simulink library "EngineModelsLibrary"  (R2014b)
settings: Solver=ode45  StartTime=0.0  StopTime=10.0  RelTol=1e-3
values from neighbouring files (symbols this model uses):
  k = 0.2    [ES_Run.m]    (also in ES_Run_v2.m = 10)
undefined symbols (not defined in the file or in its folder): b, COBRA_Compressor, cp, CPT_COBRA_LIB, D, etalim, gam, Newton, Pa, PARAM, Pl, pref, Ps, R, Raphson, rlim, T_0, Tref, Wclim
undefined symbols (not defined in the file): cr, e, etagain, fit_pars, kL, kS, par
(part 2 of 3)

== system EngineModelsLibrary/Throttle [Alt] ==
  pin (Pa) : Inport
  Tin (K) : Inport  Port=2
  pout (Pa) : Inport  Port=3
  Tout (K) : Inport  Port=4
  uth (%) : Inport  Port=5
  Compressible flow : Subsystem  mask{gam=gam, R=R, PIlin=PIlin}
      mask prompts: gam "Specific heat ratio (-)"; R "Ideal gas constant (J/kg/K)"; PIlin "Linear segment minimum pressure ratio (-)"
      mask help: Isentropic compressible flow, see App. C in Heywood (1988). Modified by adding a linear segment for pressure ratios larger than the parameter PIlin. In this way, it is possible to avoid infinite derivative for pressure ratios close to one. -- erikhe@umich
  Throttle area : Subsystem
  Wth (kg/s) : Outport
  Tth (K) : Outport  Port=2
  wires:
  uth (%)/1 -> Throttle area/1(uth (%))
  pin (Pa)/1 -> Compressible flow/1(pin (Pa))
  Tin (K)/1 -> Compressible flow/2(Tin (K))
  pout (Pa)/1 -> Compressible flow/3(pout (Pa))
  Tout (K)/1 -> Compressible flow/4(Tout (K))
  Throttle area/1(A (m^2)) -> Compressible flow/5(Aeff (m^2))
  Compressible flow/1(mflow (kg/s)) -> Wth (kg/s)/1
  Compressible flow/2(Tflow (K)) -> Tth (K)/1

== system EngineModelsLibrary/Throttle [simple] ==
  pin (Pa) : Inport
  Tin (K) : Inport  Port=2
  pout (Pa) : Inport  Port=3
  Tout (K) : Inport  Port=4
  uth (-) : Inport  Port=5
  Compressible flow : Subsystem  mask{gam=gam, R=R, PIlin=PIlin}
      mask prompts: gam "Specific heat ratio (-)"; R "Ideal gas constant (J/kg/K)"; PIlin "Linear segment minimum pressure ratio (-)"
      mask help: Isentropic compressible flow, see App. C in Heywood (1988). Modified by adding a linear segment for pressure ratios larger than the parameter PIlin. In this way, it is possible to avoid infinite derivative for pressure ratios close to one. -- erikhe@umich
  Gain : Gain  Gain=pi
  Throttle area : Subsystem
  Wth (kg/s) : Outport
  Tth (K) : Outport  Port=2
  wires:
  Compressible flow/2(Tflow (K)) -> Tth (K)/1
  Compressible flow/1(mflow (kg/s)) -> Wth (kg/s)/1
  Throttle area/1(A (m^2)) -> Compressible flow/5(Aeff (m^2))
  Tout (K)/1 -> Compressible flow/4(Tout (K))
  pout (Pa)/1 -> Compressible flow/3(pout (Pa))
  Tin (K)/1 -> Compressible flow/2(Tin (K))
  pin (Pa)/1 -> Compressible flow/1(pin (Pa))
  Gain/1 -> Throttle area/1(alpha (rad))
  uth (-)/1 -> Gain/1

== system EngineModelsLibrary/Turbine [Eriksson] ==
  pin (Pa) : Inport
  Tin (K) : Inport  Port=2
  w (rad/s) : Inport  Port=3
  pout (Pa) : Inport  Port=4
  Efficiency : Subsystem
  Mass flow : Subsystem
  Power : Subsystem
  Pressure ratio w saturation : Subsystem
  Temperature : Subsystem
  To Workspace2 : ToWorkspace  VariableName=etat  SampleTime=-1
  Tt (K) : Outport
  Wt (kg/s) : Outport  Port=2
  Pt (W) : Outport  Port=3
  wires:
  Power/1(P (W)) -> Pt (W)/1
  Pressure ratio w saturation/1(PI (-)) -> Mass flow/3(PI (-)), Efficiency/1(PI (-)), Temperature/1(PI (-))
  Tin (K)/1 -> Mass flow/2(Tin (K)), Efficiency/2(Tin (K)), Temperature/2(Tin (K)), Power/2(Tin (K))
  w (rad/s)/1 -> Efficiency/3(w (rad/s))
  Efficiency/1(etat (-)) -> To Workspace2/1, Temperature/3(etat (-))
  Temperature/1(Tout (K)) -> Power/3(Tout (K)), Tt (K)/1
  Mass flow/1(Wt (kg/s)) -> Power/1(W (kg/s)), Wt (kg/s)/1
  pin (Pa)/1 -> Mass flow/1(pin (Pa)), Pressure ratio w saturation/1(pin (Pa))
  pout (Pa)/1 -> Pressure ratio w saturation/2(pout (Pa))

== system EngineModelsLibrary/Turbine [Jensen,Moraal] ==
  pin (Pa) : Inport
  Tin (K) : Inport  Port=2
  w (rad/s) : Inport  Port=3
  pout (Pa) : Inport  Port=4
  Corrected speed : Subsystem
  Efficiency : Subsystem
  Gain : Gain  Gain=60
  Mass flow : Subsystem
  Power : Subsystem
  Pressure ratio w saturation : Subsystem
  Temperature : Subsystem
  Pt (W) : Outport
  etat (-) : Outport  Port=2
  Tt (K) : Outport  Port=3
  Wt (kg/s) : Outport  Port=4
  wires:
  w (rad/s)/1 -> Corrected speed/2(w (rad/s))
  Tin (K)/1 -> Corrected speed/1(Tin (K)), Mass flow/2(Tin (K)), Power/2(Tin (K)), Temperature/2(Tin (K))
  pin (Pa)/1 -> Mass flow/1(pin (Pa)), Pressure ratio w saturation/1(pin (Pa))
  pout (Pa)/1 -> Pressure ratio w saturation/2(pout (Pa))
  Pressure ratio w saturation/1(PI (-)) -> Temperature/1(PI (-)), Efficiency/1(PI (-)), Mass flow/3(PI (-))
  Corrected speed/1(Nc corr (rps/K^.5)) -> Gain/1
  Mass flow/1(Wt (kg/s)) -> Wt (kg/s)/1, Power/1(W (kg/s))
  Temperature/1(Tout (K)) -> Tt (K)/1, Power/3(Tout (K))
  Efficiency/1(etat (-)) -> etat (-)/1, Temperature/3(etat (-))
  Power/1(P (W)) -> Pt (W)/1
  Gain/1 -> Mass flow/4(Ncorr (rpm/K^.5)), Efficiency/2(Ncorr (rpm/K^.5))

== system EngineModelsLibrary/Turbine and wastegate ==
  note: Wastegate is a compressible flow restriction. Flows are assumed to be mixed
      | adiabatically with constant specific heat (i.e., mass-averaged temperature).
      | -- erikhe@umich
  pin (Pa) : Inport
  w (rad/s) : Inport  Port=2
  Tin (K) : Inport  Port=3
  pout (Pa) : Inport  Port=4
  uwg (%) : Inport  Port=5
  Gain : Gain  Gain=PARAM.wastegate.C
  Product : Product  RndMeth=Zero
  Product1 : Product  RndMeth=Zero
  Product2 : Product  Inputs=*/  RndMeth=Zero
  Saturation : Saturate  UpperLimit=100  LowerLimit=0
  Sum : Sum  Inputs=++|
  Sum1 : Sum
  Turbine [Jensen,Moraal] : Subsystem  mask{gam=PARAM.exh.gamma, cp=PARAM.exh.cp, D=PARAM.turbine.D, k11=PARAM.turbine.k11, k12=PARAM.turbine.k12, k21=PARAM.turbine.k21, k22=PARAM.turbine.k22, PIlin=PARAM.turbine.PIlin, Wtcmax=PARAM.turbine.Wtcmax, Wtcmin=PARAM.turbine.Wtcmin, b0=PARAM.turbine.b0, b1=PARAM.turbine.b1, b2=PARAM.turbine.b2, b3=PARAM.turbine.b3, b4=PARAM.turbine.b4, b5=PARAM.turbine.b5, etamax=PARAM.turbine.etamax, etamin=PARAM.turbine.etamin}
      mask prompts: gam "Ratio of specific heats (-)"; cp "Specific heat cp (J/kg/K)"; D "Diameter (m)"; k11 "Mass flow fit k11"; k12 "Mass flow fit k12"; k21 "Mass flow fit k21"; k22 "Mass flow fit k22"; PIlin "Mass flow PIlin"; Wtcmax "Mass flow max (kg/s K^.5/Pa)"; Wtcmin "Mass flow min (kg/s K^.5/Pa)"; b0 "Efficiency fit b0"; b1 "Efficiency fit b1"; b2 "Efficiency fit b2"; b3 "Efficiency fit b3"; b4 "Efficiency fit b4"; b5 "Efficiency fit b5"; etamax "Efficiency max (-)"; etamin "Efficiency min (-)"
  Wastegate : Subsystem  mask{gam=PARAM.exh.gamma, R=PARAM.exh.R, PIlin=PARAM.wastegate.PIlin}
      mask prompts: gam "Specific heat ratio (-)"; R "Ideal gas constant (J/kg/K)"; PIlin "Linear segment minimum pressure ratio (-)"
      mask help: Isentropic compressible flow, see App. C in Heywood (1988). Modified by adding a linear segment for pressure ratios larger than the parameter PIlin. In this way, it is possible to avoid infinite derivative for pressure ratios close to one. -- erikhe@umich
  Tout  (K) : Outport
  Wt (kg/s) : Outport  Port=2
  Wwg (kg/s) : Outport  Port=3
  Pt (W) : Outport  Port=4
  etat (-) : Outport  Port=5
  wires:
  Saturation/1 -> Gain/1
  Product2/1 -> Tout  (K)/1
  Sum1/1 -> Product2/1
  Product1/1 -> Sum1/2
  Product/1 -> Sum1/1
  Wastegate/2(Tflow (K)) -> Product1/2
  Turbine [Jensen,Moraal]/3(Tt (K)) -> Product/1
  Turbine [Jensen,Moraal]/4(Wt (kg/s)) -> Wt (kg/s)/1, Sum/1, Product/2
  Turbine [Jensen,Moraal]/1(Pt (W)) -> Pt (W)/1
  Turbine [Jensen,Moraal]/2(etat (-)) -> etat (-)/1
  Sum/1 -> Product2/2
  Wastegate/1(mflow (kg/s)) -> Wwg (kg/s)/1, Product1/1, Sum/2
  Gain/1 -> Wastegate/4(Aeff (m^2))
  uwg (%)/1 -> Saturation/1
  pout (Pa)/1 -> Wastegate/3(pout (Pa)), Turbine [Jensen,Moraal]/4(pout (Pa))
  w (rad/s)/1 -> Turbine [Jensen,Moraal]/3(w (rad/s))
  Tin (K)/1 -> Wastegate/2(Tin (K)), Turbine [Jensen,Moraal]/2(Tin (K))
  pin (Pa)/1 -> Wastegate/1(pin (Pa)), Turbine [Jensen,Moraal]/1(pin (Pa))

== system EngineModelsLibrary/Twin-Scroll Turbine ==
  Pems (Pa) : Inport
  Peml (Pa) : Inport  Port=2
  Pex (Pa) : Inport  Port=3
  omega (rad/s) : Inport  Port=4
  Tems (K) : Inport  Port=5
  Teml (K) : Inport  Port=6
  Demux : Demux  Outputs=5
  Mux : Mux  Inputs=6
  S-Function : S-Function  FunctionName=turbine  Parameters=eta,gam,cp,smar_fit,smar_lim,flow_fit,flow_lim  SFunctionModules=turbine engine_model  EnableBusSupport=off
  Power (W) : Outport
  Wtl (kg/s) : Outport  Port=2
  Wts (kg/s) : Outport  Port=3
  Temp (K) : Outport  Port=4
  SMaR (-) : Outport  Port=5
  wires:
  Demux/1 -> Power (W)/1
  Pems (Pa)/1 -> Mux/1
  Peml (Pa)/1 -> Mux/2
  Pex (Pa)/1 -> Mux/3
  omega (rad/s)/1 -> Mux/4
  Mux/1 -> S-Function/1
  S-Function/1 -> Demux/1
  Demux/2 -> Wtl (kg/s)/1
  Tems (K)/1 -> Mux/5
  Teml (K)/1 -> Mux/6
  Demux/3 -> Wts (kg/s)/1
  Demux/4 -> Temp (K)/1
  Demux/5 -> SMaR (-)/1

== system EngineModelsLibrary/Wastegate Area  ==
  u-u_crit (%) : Inport
  Constant : Constant  Value=c(4)
  Constant1 : Constant  Value=c(1)
  Gain : Gain  Gain=c(3)
  Gain1 : Gain  Gain=c(2)
  Gain2 : Gain  Gain=1e-4
  Gain3 : Gain  Gain=(7.3156e-5)/5
  Saturation : Saturate  UpperLimit=inf  LowerLimit=0
  Sum : Sum  Inputs=|+-
  Sum1 : Sum  Inputs=|++
  Switch : Switch  Threshold=5
  Trigonometric Function : Trigonometry  Operator=tanh
  A (m^2) : Outport
  wires:
  Saturation/1 -> Switch/3
  Gain3/1 -> Saturation/1
  Gain2/1 -> Switch/1
  Switch/1 -> A (m^2)/1
  Sum1/1 -> Gain2/1
  Constant1/1 -> Sum1/2
  Gain1/1 -> Sum1/1
  Trigonometric Function/1 -> Gain1/1
  Gain/1 -> Trigonometric Function/1
  Sum/1 -> Gain/1
  Constant/1 -> Sum/2
  u-u_crit (%)/1 -> Sum/1, Switch/2, Gain3/1

== system EngineModelsLibrary/Wastegate Flow  ==
  note: u_crit
  u_wg (-) : Inport
  P_emr (Pa) : Inport  Port=2
  P_ex (Pa) : Inport  Port=3
  T_em(K) : Inport  Port=4
  Add2 : Sum  Inputs=+-
  Constant4 : Constant  Value=0
  Constant5 : Constant  Value=R
  Convert to % : Gain  Gain=100
  Divide2 : Product  Inputs=*/
  Divide3 : Product  Inputs=***/
  Gain : Gain  Gain=par.tc.wg.gain_tune
  Get Critical WG signal : Subsystem
  Orifice flow : Subsystem
  Product1 : Product  RndMeth=Zero
  Sqrt1 : Sqrt  SaturateOnIntegerOverflow=on
  Switch : Switch
  "Wastegate Area " : Subsystem  mask{c=par.tc.wg.Area_coeff}
      mask prompts: c "Area fit functions (4 params)"
  W_wg (kg/s) : Outport
  tag scope: u_crit=global
  wires:
  Gain/1 -> [W_open]
  P_emr (Pa)/1 -> Divide2/2, Get Critical WG signal/1(P_emr (Pa)), Divide3/1
  Get Critical WG signal/1(u_crit (-)) -> Add2/2, [u_crit]
  "Wastegate Area "/1(A (m^2)) -> Divide3/2
  Convert to %/1 -> "Wastegate Area "/1(u-u_crit (%))
  Sqrt1/1 -> Divide3/4
  Product1/1 -> Sqrt1/1
  T_em(K)/1 -> Product1/2
  Constant5/1 -> Product1/1
  Divide3/1 -> Gain/1
  Orifice flow/1(Psi (-)) -> Divide3/3  "Psi"
  Divide2/1 -> "Wastegate Area "/2(Pressure ratio (-)), Orifice flow/1(Pi_wg (-))
  [W_open] -> Switch/1
  Switch/1 -> W_wg (kg/s)/1
  Add2/1 -> Switch/2, Convert to %/1
  u_wg (-)/1 -> Add2/1
  Constant4/1 -> Switch/3
  P_ex (Pa)/1 -> Divide2/1, Get Critical WG signal/2(P_ex (Pa))

== system EngineModelsLibrary/Compressor [Eriksson]/Corrected flow inv (unit preserving) ==
  note: Mass flow corrected based on inlet conditions and reference state.
      | -- erikhe@umich
  Wcorr (kg/s) : Inport
  pin (Pa) : Inport  Port=2
  Tin (K) : Inport  Port=3
  Constant : Constant  Value=Tref
  Constant2 : Constant  Value=pref
  Divide : Product  Inputs=*/
  Divide2 : Product  Inputs=*/
  Divide3 : Product  Inputs=/**
  Math Function : Math  Operator=sqrt  SaturateOnIntegerOverflow=on
  W (kg/s) : Outport
  wires:
  Divide/1 -> Math Function/1
  Constant/1 -> Divide/2
  Tin (K)/1 -> Divide/1
  Math Function/1 -> Divide3/1
  Constant2/1 -> Divide2/2
  pin (Pa)/1 -> Divide2/1
  Divide2/1 -> Divide3/3
  Wcorr (kg/s)/1 -> Divide3/2
  Divide3/1 -> W (kg/s)/1

== system EngineModelsLibrary/Compressor [Eriksson]/Corrected speed ==
  note: Speed corrected based on inlet conditions and reference state.
      | -- erikhe@umich
  w (rad/s) : Inport
  Tin (K) : Inport  Port=2
  Constant : Constant  Value=Tref
  Divide : Product  Inputs=*/
  Divide1 : Product  Inputs=*/
  Gain1 : Gain  Gain=1/(2*pi)
  Math Function : Math  Operator=sqrt  SaturateOnIntegerOverflow=on
  Ncorr (rps) : Outport
  wires:
  Tin (K)/1 -> Divide/1
  Gain1/1 -> Divide1/1
  Divide1/1 -> Ncorr (rps)/1
  Math Function/1 -> Divide1/2
  Constant/1 -> Divide/2
  Divide/1 -> Math Function/1
  w (rad/s)/1 -> Gain1/1

== system EngineModelsLibrary/Compressor [Eriksson]/Density ==
  p (Pa) : Inport
  T (K) : Inport  Port=2
  Constant1 : Constant  Value=R
  Product : Product  Inputs=*//  RndMeth=Zero
  rho (kg/m^3) : Outport
  wires:
  Product/1 -> rho (kg/m^3)/1
  Constant1/1 -> Product/3
  T (K)/1 -> Product/2
  p (Pa)/1 -> Product/1

== system EngineModelsLibrary/Compressor [Eriksson]/Efficiency ==
  note: Semi-physical model of compressor efficiency, see e.g. Eriksson (2007)
      | Modeling and control of turbocharged SI and DI engines, Oil&Gas Science and Technology. -- erikhe@umich
  Wcorr (kg/s) : Inport
  rho (kg/m^3) : Inport  Port=2
  Ncorr (rps) : Inport  Port=3
  Constant1 : Constant  Value=Phimax
  Constant2 : Constant  Value=Ncorrmax
  Constant3 : Constant  Value=Q
  Constant4 : Constant  Value=etamax
  Constant6 : Constant  Value=D*D*D
  Math Function : Math  Operator=transpose  SaturateOnIntegerOverflow=on
  Matrix Concatenate : Concatenate  Mode=Multidimensional array
  Product : Product  Inputs=3  Multiplication=Matrix(*)  RndMeth=Zero
  Product2 : Product  Inputs=*///  RndMeth=Zero
  Reshape : Reshape
  Saturation : Saturate  UpperLimit=etamax  LowerLimit=etamin
  Sum : Sum  Inputs=|+-
  Sum1 : Sum  Inputs=|+-
  Sum2 : Sum  Inputs=|+-
  etac (-) : Outport
  wires:
  Ncorr (rps)/1 -> Sum1/1, Product2/3
  Reshape/1 -> Sum2/2
  Constant6/1 -> Product2/4
  Wcorr (kg/s)/1 -> Product2/1
  Product2/1 -> Sum/1  "Phi"
  rho (kg/m^3)/1 -> Product2/2
  Constant1/1 -> Sum/2
  Constant2/1 -> Sum1/2
  Sum/1 -> Matrix Concatenate/1
  Sum1/1 -> Matrix Concatenate/2
  Matrix Concatenate/1 -> Math Function/1, Product/3  "Chi"
  Math Function/1 -> Product/1
  Constant3/1 -> Product/2
  Product/1 -> Reshape/1
  Constant4/1 -> Sum2/1
  Sum2/1 -> Saturation/1
  Saturation/1 -> etac (-)/1

== system EngineModelsLibrary/Compressor [Eriksson]/Mass flow ==
  note: Semi-physical model of compressor mass flow, see e.g. Eriksson (2007)
      | Modeling and control of turbocharged SI and DI engines, Oil&Gas Science and Technology. -- erikhe@umich
  Ncorr (rps) : Inport
  PI (-) : Inport  Port=2
  pin (Pa) : Inport  Port=3
  Tin (K) : Inport  Port=4
  Constant : Constant  Value=1-1/gam
  Constant1 : Constant
  Constant2 : Constant  Value=8*cp/(D*D)
  Constant3 : Constant  Value=a2
  Constant4 : Constant
  Constant5 : Constant  Value=0
  Constant6 : Constant  Value=D*D*D
  Density : Subsystem
  Gain : Gain  Gain=a1
  Gain1 : Gain  Gain=2*pi
  Math Function : Math  Operator=pow  SaturateOnIntegerOverflow=on
  Math Function1 : Math  Operator=sqrt  SaturateOnIntegerOverflow=on
  MinMax : MinMax  Function=max  Inputs=2
  Product : Product  Inputs=*//**  RndMeth=Zero
  Product1 : Product  Inputs=**//  RndMeth=Zero
  Product2 : Product  Inputs=4  RndMeth=Zero
  Sum : Sum  Inputs=|+-
  Sum1 : Sum  Inputs=|-+
  Wcorr (kg/s) : Outport
  wires:
  Gain1/1 -> Product/3, Product/2
  pin (Pa)/1 -> Density/1(p (Pa))
  Tin (K)/1 -> Density/2(T (K)), Product/1
  PI (-)/1 -> Math Function/1
  Constant/1 -> Math Function/2
  Math Function/1 -> Sum/1
  Constant1/1 -> Sum/2
  Ncorr (rps)/1 -> Gain1/1, Product2/2
  Sum/1 -> Product/4
  Constant2/1 -> Product/5
  Product/1 -> Product1/1, Product1/2  "Psi"
  Constant3/1 -> Product1/3, Product1/4
  Product1/1 -> Sum1/1
  Constant4/1 -> Sum1/2
  Sum1/1 -> MinMax/1
  Constant5/1 -> MinMax/2
  MinMax/1 -> Math Function1/1
  Math Function1/1 -> Gain/1
  Gain/1 -> Product2/3  "Phi"
  Constant6/1 -> Product2/4
  Product2/1 -> Wcorr (kg/s)/1
  Density/1(rho (kg/m^3)) -> Product2/1

== system EngineModelsLibrary/Compressor [Eriksson]/Power ==
  W (kg/s) : Inport
  Tin (K) : Inport  Port=2
  Tout (K) : Inport  Port=3
  Constant : Constant  Value=cp
  Product : Product  Inputs=3  RndMeth=Zero
  Sum : Sum  Inputs=|-+
  P (W) : Outport
  wires:
  Tout (K)/1 -> Sum/2
  Tin (K)/1 -> Sum/1
  Constant/1 -> Product/3
  W (kg/s)/1 -> Product/1
  Sum/1 -> Product/2
  Product/1 -> P (W)/1

== system EngineModelsLibrary/Compressor [Eriksson]/Pressure ratio ==
  pin (Pa) : Inport
  pout (Pa) : Inport  Port=2
  Constant : Constant
  Divide : Product  Inputs=*/
  MinMax : MinMax  Function=max  Inputs=2
  PI (-) : Outport
  wires:
  pout (Pa)/1 -> Divide/1
  pin (Pa)/1 -> Divide/2
  Divide/1 -> MinMax/1
  Constant/1 -> MinMax/2
  MinMax/1 -> PI (-)/1

== system EngineModelsLibrary/Compressor [Eriksson]/Temperature ==
  note: Temperature solved from the definition of efficiency. -- erikhe@umich
  Tin (K) : Inport
  PI (-) : Inport  Port=2
  etac (-) : Inport  Port=3
  Constant1 : Constant  Value=1-1/gam
  Constant2 : Constant
  Divide : Product  Inputs=*/
  Divide1 : Product  Inputs=**
  Math Function : Math  Operator=pow  SaturateOnIntegerOverflow=on
  Sum : Sum  Inputs=-+|
  Sum1 : Sum  Inputs=++|
  Tout (K) : Outport
  wires:
  PI (-)/1 -> Math Function/1
  Constant1/1 -> Math Function/2
  Sum/1 -> Divide/1
  etac (-)/1 -> Divide/2
  Sum1/1 -> Divide1/2
  Tin (K)/1 -> Divide1/1
  Divide1/1 -> Tout (K)/1
  Math Function/1 -> Sum/2
  Constant2/1 -> Sum/1, Sum1/1
  Divide/1 -> Sum1/2

== system EngineModelsLibrary/Compressor [Jensen simplified]/Corrected flow inv (unit preserving) ==
  note: Mass flow corrected based on inlet conditions and reference state.
      | -- erikhe@umich
  Wcorr (kg/s) : Inport
  pin (Pa) : Inport  Port=2
  Tin (K) : Inport  Port=3
  Constant : Constant  Value=Tref
  Constant2 : Constant  Value=pref
  Divide : Product  Inputs=*/
  Divide2 : Product  Inputs=*/
  Divide3 : Product  Inputs=/**
  Math Function : Math  Operator=sqrt  SaturateOnIntegerOverflow=on
  W (kg/s) : Outport
  wires:
  Divide3/1 -> W (kg/s)/1
  Wcorr (kg/s)/1 -> Divide3/2
  Divide2/1 -> Divide3/3
  pin (Pa)/1 -> Divide2/1
  Constant2/1 -> Divide2/2
  Math Function/1 -> Divide3/1
  Tin (K)/1 -> Divide/1
  Constant/1 -> Divide/2
  Divide/1 -> Math Function/1

== system EngineModelsLibrary/Compressor [Jensen simplified]/Corrected speed ==
  note: Speed corrected based on inlet conditions and reference state.
      | -- erikhe@umich
  w (rad/s) : Inport
  Tin (K) : Inport  Port=2
  Constant : Constant  Value=Tref
  Divide : Product  Inputs=*/
  Divide1 : Product  Inputs=*/
  Gain1 : Gain  Gain=1/(2*pi)
  Math Function : Math  Operator=sqrt  SaturateOnIntegerOverflow=on
  Ncorr (rps) : Outport
  wires:
  w (rad/s)/1 -> Gain1/1
  Divide/1 -> Math Function/1
  Constant/1 -> Divide/2
  Math Function/1 -> Divide1/2
  Divide1/1 -> Ncorr (rps)/1
  Gain1/1 -> Divide1/1
  Tin (K)/1 -> Divide/1

== system EngineModelsLibrary/Compressor [Jensen simplified]/Density ==
  p (Pa) : Inport
  T (K) : Inport  Port=2
  Constant1 : Constant  Value=R
  Product : Product  Inputs=*//  RndMeth=Zero
  rho (kg/m^3) : Outport
  wires:
  p (Pa)/1 -> Product/1
  T (K)/1 -> Product/2
  Constant1/1 -> Product/3
  Product/1 -> rho (kg/m^3)/1

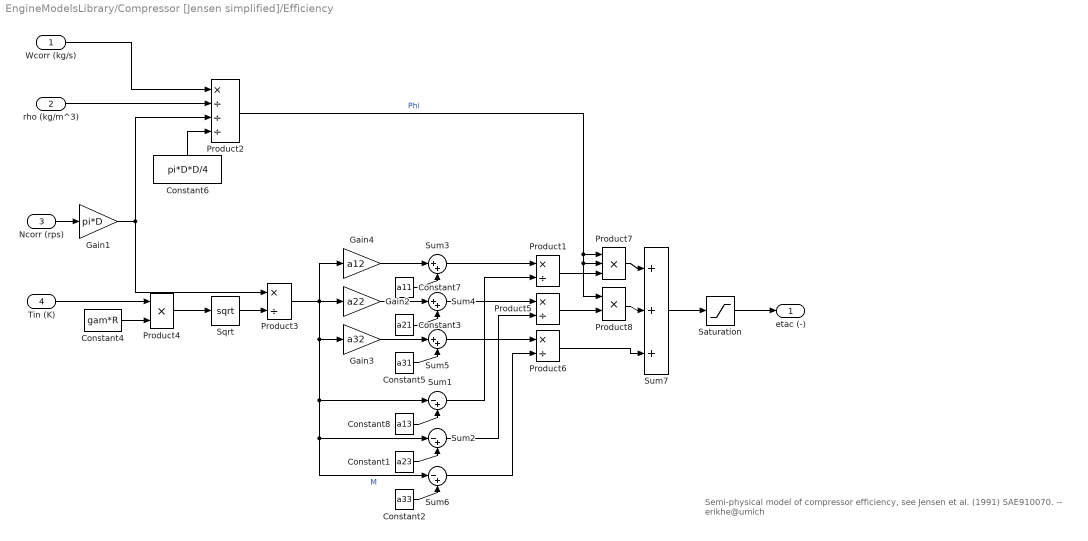
== system EngineModelsLibrary/Compressor [Jensen simplified]/Efficiency ==
  note: Semi-physical model of compressor efficiency, see Jensen et al. (1991) SAE910070.
      | -- erikhe@umich
  Wcorr (kg/s) : Inport
  rho (kg/m^3) : Inport  Port=2
  Ncorr (rps) : Inport  Port=3
  Tin (K) : Inport  Port=4
  Constant1 : Constant  Value=a23
  Constant2 : Constant  Value=a33
  Constant3 : Constant  Value=a21
  Constant4 : Constant  Value=gam*R
  Constant5 : Constant  Value=a31
  Constant6 : Constant  Value=pi*D*D/4
  Constant7 : Constant  Value=a11
  Constant8 : Constant  Value=a13
  Gain1 : Gain  Gain=pi*D
  Gain2 : Gain  Gain=a22
  Gain3 : Gain  Gain=a32
  Gain4 : Gain  Gain=a12
  Product{1,3,5..6} (4 alike) : Product  Inputs=*/  RndMeth=Zero
  Product2 : Product  Inputs=*///  RndMeth=Zero
  Product4 : Product  RndMeth=Zero
  Product7 : Product  Inputs=3  RndMeth=Zero
  Product8 : Product  RndMeth=Zero
  Saturation : Saturate  UpperLimit=etamax  LowerLimit=etamin
  Sqrt : Sqrt  AlgorithmType=Newton-Raphson  SaturateOnIntegerOverflow=on
  Sum1 : Sum  Inputs=|-+
  Sum2 : Sum  Inputs=|-+
  Sum3 : Sum  Inputs=|++
  Sum4 : Sum  Inputs=|++
  Sum5 : Sum  Inputs=|++
  Sum6 : Sum  Inputs=|-+
  Sum7 : Sum  Inputs=3
  etac (-) : Outport
  wires:
  Sum7/1 -> Saturation/1
  Product7/1 -> Sum7/1
  Product8/1 -> Sum7/2
  Product6/1 -> Sum7/3
  Product5/1 -> Product8/2
  Product1/1 -> Product7/3
  Product2/1 -> Product8/1, Product7/2, Product7/1  "Phi"
  Sum6/1 -> Product6/2
  Sum5/1 -> Product6/1
  Sum2/1 -> Product5/2
  Sum4/1 -> Product5/1
  Sum1/1 -> Product1/2
  Sum3/1 -> Product1/1
  Constant2/1 -> Sum6/2
  Constant1/1 -> Sum2/2
  Constant8/1 -> Sum1/2
  Tin (K)/1 -> Product4/1
  Constant5/1 -> Sum5/2
  Constant3/1 -> Sum4/2
  Constant7/1 -> Sum3/2
  Gain3/1 -> Sum5/1
  Gain2/1 -> Sum4/1
  Gain4/1 -> Sum3/1
  Product3/1 -> Sum6/1, Sum2/1, Sum1/1, Gain3/1, Gain4/1, Gain2/1  "M"
  Constant4/1 -> Product4/2
  Product4/1 -> Sqrt/1
  Sqrt/1 -> Product3/2
  Gain1/1 -> Product3/1, Product2/3
  Ncorr (rps)/1 -> Gain1/1
  Saturation/1 -> etac (-)/1
  rho (kg/m^3)/1 -> Product2/2
  Wcorr (kg/s)/1 -> Product2/1
  Constant6/1 -> Product2/4

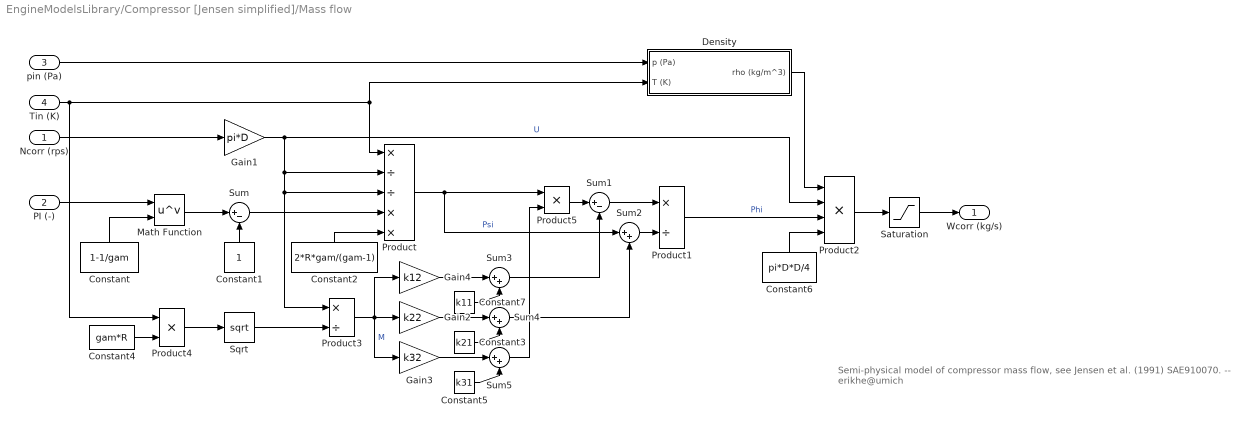
== system EngineModelsLibrary/Compressor [Jensen simplified]/Mass flow ==
  note: Semi-physical model of compressor mass flow, see Jensen et al. (1991) SAE910070.
      | -- erikhe@umich
  Ncorr (rps) : Inport
  PI (-) : Inport  Port=2
  pin (Pa) : Inport  Port=3
  Tin (K) : Inport  Port=4
  Constant : Constant  Value=1-1/gam
  Constant1 : Constant
  Constant2 : Constant  Value=2*R*gam/(gam-1)
  Constant3 : Constant  Value=k21
  Constant4 : Constant  Value=gam*R
  Constant5 : Constant  Value=k31
  Constant6 : Constant  Value=pi*D*D/4
  Constant7 : Constant  Value=k11
  Density : Subsystem
  Gain1 : Gain  Gain=pi*D
  Gain2 : Gain  Gain=k22
  Gain3 : Gain  Gain=k32
  Gain4 : Gain  Gain=k12
  Math Function : Math  Operator=pow  SaturateOnIntegerOverflow=on
  Product : Product  Inputs=*//**  RndMeth=Zero
  Product1 : Product  Inputs=*/  RndMeth=Zero
  Product2 : Product  Inputs=4  RndMeth=Zero
  Product3 : Product  Inputs=*/  RndMeth=Zero
  Product4 : Product  RndMeth=Zero
  Product5 : Product  RndMeth=Zero
  Saturation : Saturate  UpperLimit=Wcmax  LowerLimit=Wcmin
  Sqrt : Sqrt  AlgorithmType=Newton-Raphson  SaturateOnIntegerOverflow=on
  Sum : Sum  Inputs=|+-
  Sum1 : Sum  Inputs=|+-
  Sum{2..5} (4 alike) : Sum  Inputs=|++
  Wcorr (kg/s) : Outport
  wires:
  Sum5/1 -> Product5/2
  Sum3/1 -> Sum1/2
  Sum4/1 -> Sum2/2
  Product5/1 -> Sum1/1
  Constant5/1 -> Sum5/2
  Constant3/1 -> Sum4/2
  Constant7/1 -> Sum3/2
  Gain3/1 -> Sum5/1
  Gain2/1 -> Sum4/1
  Gain4/1 -> Sum3/1
  Product3/1 -> Gain3/1, Gain4/1, Gain2/1  "M"
  Constant4/1 -> Product4/2
  Product4/1 -> Sqrt/1
  Sqrt/1 -> Product3/2
  Gain1/1 -> Product2/2, Product3/1, Product/3, Product/2  "U"
  Sum2/1 -> Product1/2
  Sum1/1 -> Product1/1
  Density/1(rho (kg/m^3)) -> Product2/1
  Product2/1 -> Saturation/1
  Constant6/1 -> Product2/4
  Product1/1 -> Product2/3  "Phi"
  Product/1 -> Product5/1, Sum2/1  "Psi"
  Constant2/1 -> Product/5
  Sum/1 -> Product/4
  Ncorr (rps)/1 -> Gain1/1
  Constant1/1 -> Sum/2
  Math Function/1 -> Sum/1
  Constant/1 -> Math Function/2
  PI (-)/1 -> Math Function/1
  Tin (K)/1 -> Product4/1, Product/1, Density/2(T (K))
  pin (Pa)/1 -> Density/1(p (Pa))
  Saturation/1 -> Wcorr (kg/s)/1

== system EngineModelsLibrary/Compressor [Jensen simplified]/Power ==
  W (kg/s) : Inport
  Tin (K) : Inport  Port=2
  Tout (K) : Inport  Port=3
  Constant : Constant  Value=R*gam/(gam-1)
  Product : Product  Inputs=3  RndMeth=Zero
  Sum : Sum  Inputs=|-+
  P (W) : Outport
  wires:
  Product/1 -> P (W)/1
  Sum/1 -> Product/2
  W (kg/s)/1 -> Product/1
  Constant/1 -> Product/3
  Tin (K)/1 -> Sum/1
  Tout (K)/1 -> Sum/2

== system EngineModelsLibrary/Compressor [Jensen simplified]/Pressure ratio ==
  pin (Pa) : Inport
  pout (Pa) : Inport  Port=2
  Constant : Constant
  Divide : Product  Inputs=*/
  MinMax : MinMax  Function=max  Inputs=2
  PI (-) : Outport
  wires:
  MinMax/1 -> PI (-)/1
  Constant/1 -> MinMax/2
  Divide/1 -> MinMax/1
  pin (Pa)/1 -> Divide/2
  pout (Pa)/1 -> Divide/1

== system EngineModelsLibrary/Compressor [Jensen simplified]/Temperature ==
  note: Temperature solved from the definition of efficiency. -- erikhe@umich
  Tin (K) : Inport
  PI (-) : Inport  Port=2
  etac (-) : Inport  Port=3
  Constant1 : Constant  Value=1-1/gam
  Constant2 : Constant
  Divide : Product  Inputs=*/
  Divide1 : Product  Inputs=**
  Math Function : Math  Operator=pow  SaturateOnIntegerOverflow=on
  Sum : Sum  Inputs=-+|
  Sum1 : Sum  Inputs=++|
  Tout (K) : Outport
  wires:
  Divide/1 -> Sum1/2
  Constant2/1 -> Sum1/1, Sum/1
  Math Function/1 -> Sum/2
  Divide1/1 -> Tout (K)/1
  Tin (K)/1 -> Divide1/1
  Sum1/1 -> Divide1/2
  etac (-)/1 -> Divide/2
  Sum/1 -> Divide/1
  Constant1/1 -> Math Function/2
  PI (-)/1 -> Math Function/1

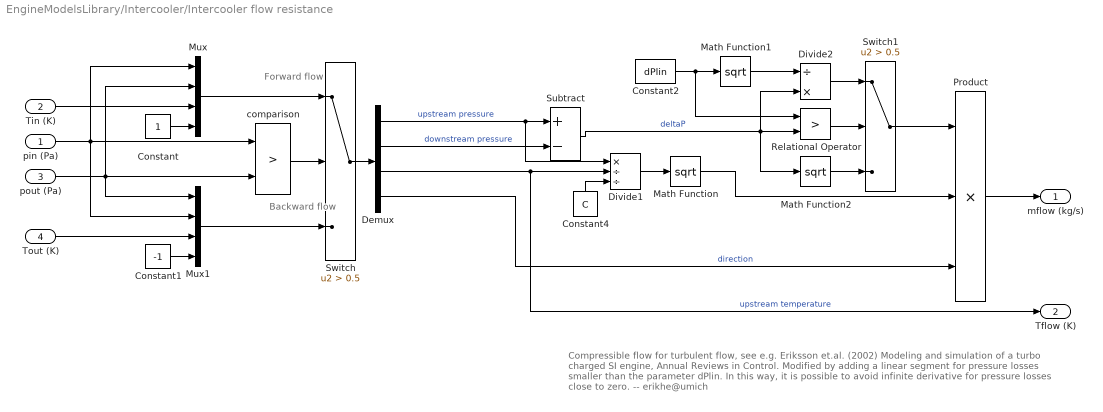
== system EngineModelsLibrary/Intercooler/Intercooler flow resistance ==
  note: Compressible flow for turbulent flow, see e.g. Eriksson et.al. (2002) Modeling and simulation of a turbo charged SI engine,
      | Annual Reviews in Control. Modified by adding a linear segment for pressure losses smaller than the parameter dPlin.
      | In this way, it is possible to avoid infinite derivative for pressure losses close to zero. -- erikhe@umich
  note: Forward flow
  note: Backward flow
  pin (Pa) : Inport
  Tin (K) : Inport  Port=2
  pout (Pa) : Inport  Port=3
  Tout (K) : Inport  Port=4
  Constant : Constant
  Constant1 : Constant  Value=-1
  Constant2 : Constant  Value=dPlin
  Constant4 : Constant  Value=C
  Demux : Demux
  Divide1 : Product  Inputs=*//
  Divide2 : Product  Inputs=/*
  Math Function : Math  Operator=sqrt  SaturateOnIntegerOverflow=on
  Math Function1 : Math  Operator=sqrt  SaturateOnIntegerOverflow=on
  Math Function2 : Math  Operator=sqrt  SaturateOnIntegerOverflow=on
  Mux : Mux
  Mux1 : Mux
  Product : Product  Inputs=3  RndMeth=Zero
  Relational Operator : RelationalOperator  Operator=>  OutDataTypeStr=boolean
  Subtract : Sum  Inputs=+-
  Switch : Switch  Criteria=u2 > Threshold  Threshold=0.5
  Switch1 : Switch  Criteria=u2 > Threshold  Threshold=0.5
  comparison : RelationalOperator  Operator=>  OutDataTypeStr=boolean
  mflow (kg/s) : Outport
  Tflow (K) : Outport  Port=2
  wires:
  Switch1/1 -> Product/1
  Math Function2/1 -> Switch1/3
  Math Function1/1 -> Divide2/1
  Divide2/1 -> Switch1/1
  Constant2/1 -> Math Function1/1, Relational Operator/1
  Relational Operator/1 -> Switch1/2
  Math Function/1 -> Product/2
  Divide1/1 -> Math Function/1
  Constant4/1 -> Divide1/3
  Subtract/1 -> Math Function2/1, Divide2/2, Relational Operator/2  "deltaP"
  Product/1 -> mflow (kg/s)/1
  Demux/4 -> Product/3  "direction"
  Constant1/1 -> Mux1/4
  Constant/1 -> Mux/4
  Demux/3 -> Divide1/2, Tflow (K)/1  "upstream temperature"
  Demux/2 -> Subtract/2  "downstream pressure"
  Demux/1 -> Divide1/1, Subtract/1  "upstream pressure"
  Switch/1 -> Demux/1
  Tout (K)/1 -> Mux1/3
  Tin (K)/1 -> Mux/3
  Mux1/1 -> Switch/3
  Mux/1 -> Switch/1
  pout (Pa)/1 -> comparison/2, Mux/2, Mux1/1
  pin (Pa)/1 -> Mux1/2, comparison/1, Mux/1
  comparison/1 -> Switch/2

== system EngineModelsLibrary/Intercooler/Intercooler temperature ==
  note: Intercooler temperature model, see e.g. Eriksson et al. (2002)
      | Modeling of a turbocharged SI engine, Annual reviews in Control.
      | -- erikhe@umich
  Tco (K) : Inport
  Win (kg/s) : Inport  Port=2
  Tin (K) : Inport  Port=3
  Constant : Constant  Value=a0
  Gain : Gain  Gain=a1
  Gain1 : Gain  Gain=a2
  Gain2 : Gain  Gain=.5
  Product : Product  RndMeth=Zero
  Saturation : Saturate  UpperLimit=1  LowerLimit=0
  Sum : Sum  Inputs=2
  Sum1 : Sum  Inputs=+++
  Sum2 : Sum  Inputs=+-
  Sum3 : Sum  Inputs=+-|
  Tic (K) : Outport
  wires:
  Saturation/1 -> Product/2
  Sum3/1 -> Tic (K)/1
  Product/1 -> Sum3/2
  Tin (K)/1 -> Sum3/1, Sum/1, Sum2/1
  Tco (K)/1 -> Sum/2, Sum2/2
  Sum/1 -> Gain2/1
  Gain2/1 -> Gain1/1
  Win (kg/s)/1 -> Gain/1
  Constant/1 -> Sum1/1
  Gain1/1 -> Sum1/2
  Gain/1 -> Sum1/3
  Sum1/1 -> Saturation/1  "efficiency"
  Sum2/1 -> Product/1

== system EngineModelsLibrary/Jensen Compressor Flow /Density ==
  p (Pa) : Inport
  T (K) : Inport  Port=2
  Constant1 : Constant  Value=R
  Product : Product  Inputs=*//  RndMeth=Zero
  rho (kg/m^3) : Outport
  wires:
  Product/1 -> rho (kg/m^3)/1
  Constant1/1 -> Product/3
  T (K)/1 -> Product/2
  p (Pa)/1 -> Product/1

== system EngineModelsLibrary/Jensen Compressor Flow /Saturate PI ==
  note: Saturate the pressure ratio at the value where the model for normalized flow (PhI) crosses zero.
  U : Inport
  PI : Inport  Port=2
  K1 : Inport  Port=3
  K3 : Inport  Port=4
  Constant : Constant  Value=gam/(gam-1)
  Constant1 : Constant
  Gain : Gain  Gain=2*(R*gam/(gam-1))*Tref
  Math Function : Math  Operator=pow  SaturateOnIntegerOverflow=on
  MinMax : MinMax  Inputs=2
  Product : Product  Inputs=3  RndMeth=Zero
  Product1 : Product  Inputs=*/  RndMeth=Zero
  Sum : Sum  Inputs=|++
  PIsat : Outport
  wires:
  K3/1 -> Gain/1
  K1/1 -> Product/3
  U/1 -> Product/2, Product/1
  Product/1 -> Product1/1
  Gain/1 -> Product1/2
  Constant1/1 -> Sum/2
  Product1/1 -> Sum/1
  Sum/1 -> Math Function/1
  Constant/1 -> Math Function/2
  Math Function/1 -> MinMax/2
  PI/1 -> MinMax/1
  MinMax/1 -> PIsat/1

== system EngineModelsLibrary/Jensen Compressor Flow /Saturation ==
  u : Inport
  Assertion : Assertion  StopWhenAssertionFail=off
  Relational Operator : RelationalOperator  Operator===  OutDataTypeStr=boolean
  Saturation : Saturate  UpperLimit=lim(2)  LowerLimit=lim(1)
  Sat(u) : Outport
  wires:
  Saturation/1 -> Sat(u)/1, Relational Operator/2
  u/1 -> Saturation/1, Relational Operator/1
  Relational Operator/1 -> Assertion/1

== system EngineModelsLibrary/Large scroll turbine/Mass flow ==
  note: Empirical model of turbine mass flow, see e.g. Eriksson (2007)
      | Modeling and control of turbocharged SI and DI engines, Oil&Gas Science and Technology.
      | Extended by letting the two parameters depend on the mach number ratio r.
      | -- erikhe@umich
  r (-) : Inport
  Pin (Pa) : Inport  Port=2
  Tin (K) : Inport  Port=3
  PI (-) : Inport  Port=4
  Constant1 : Constant  Value=k(3)
  Constant2 : Constant
  Constant3 : Constant  Value=k(4)
  Constant4 : Constant  Value=k(1)
  Constant5 : Constant  Value=0
  Constant6 : Constant  Value=k(2)
  Corrected flow inv : Subsystem
  Gain : Gain  Gain=1e-5
  Math Function : Math  Operator=pow  SaturateOnIntegerOverflow=on
  Math Function1 : Math  Operator=sqrt  SaturateOnIntegerOverflow=on
  MinMax : MinMax  Function=max  Inputs=2
  Product1 : Product  RndMeth=Zero
  Product2 : Product  RndMeth=Zero
  Product3 : Product  RndMeth=Zero
  Saturation : Saturate  UpperLimit=Wclim(2)  LowerLimit=Wclim(1)
  Sum : Sum  Inputs=|-+
  Sum1 : Sum  Inputs=|++
  Sum2 : Sum  Inputs=|++
  Wt (kg/s) : Outport
  wires:
  Saturation/1 -> Corrected flow inv/3(Wt corr (kg/s K^.5/bar))
  Gain/1 -> Corrected flow inv/1(Pin (bar))
  Constant6/1 -> Product2/2
  Product2/1 -> Sum2/1
  Constant4/1 -> Sum2/2
  Sum2/1 -> Product1/2
  r (-)/1 -> Product2/1, Product3/1
  Constant3/1 -> Product3/2
  Product3/1 -> Sum1/1
  Constant1/1 -> Sum1/2
  Sum1/1 -> Math Function/2
  Corrected flow inv/1(Wt (kg/s)) -> Wt (kg/s)/1
  Sum/1 -> MinMax/1
  MinMax/1 -> Math Function1/1
  Constant5/1 -> MinMax/2
  PI (-)/1 -> Math Function/1
  Math Function/1 -> Sum/1
  Constant2/1 -> Sum/2
  Pin (Pa)/1 -> Gain/1
  Tin (K)/1 -> Corrected flow inv/2(Tin (K))
  Math Function1/1 -> Product1/1
  Product1/1 -> Saturation/1

== system EngineModelsLibrary/Mass flow/Corrected flow inv ==
  note: Inversion of mass flow corrected based on inlet conditions.
      | -- erikhe@umich
  Pin (bar) : Inport
  Tin (K) : Inport  Port=2
  Wt corr (kg/s K^.5/bar) : Inport  Port=3
  Divide3 : Product  Inputs=/**
  Math Function : Math  Operator=sqrt  SaturateOnIntegerOverflow=on
  Wt (kg/s) : Outport
  wires:
  Divide3/1 -> Wt (kg/s)/1
  Wt corr (kg/s K^.5/bar)/1 -> Divide3/2
  Pin (bar)/1 -> Divide3/3
  Math Function/1 -> Divide3/1
  Tin (K)/1 -> Math Function/1

== system EngineModelsLibrary/Power/Efficiency ==
  note: Empirical model of turbine efficiency,
      | a second order polynomial in BSR
      |  -- erikhe@umich
  PI (-) : Inport
  Ncorr (rps) : Inport  Port=2
  Constant : Constant  Value=1-1/gam
  Constant1 : Constant  Value=2*cp*Tref
  Constant2 : Constant
  Constant3 : Constant  Value=pi*D
  Constant4 : Constant  Value=1e-6
  Gain : Gain  Gain=gain
  Math Function : Math  Operator=pow  SaturateOnIntegerOverflow=on
  Math Function1 : Math  Operator=sqrt  SaturateOnIntegerOverflow=on
  MinMax : MinMax  Function=max  Inputs=2
  Polynomial : Polyval  Coefs=b
  Product : Product  RndMeth=Zero
  Product1 : Product  Inputs=*/*  RndMeth=Zero
  Saturation : Saturate  UpperLimit=etalim(2)  LowerLimit=etalim(1)
  Sum : Sum  Inputs=|-+
  etat (-) : Outport
  wires:
  Sum/1 -> Product/1
  Constant/1 -> Math Function/2
  PI (-)/1 -> Math Function/1
  Math Function/1 -> Sum/1
  Constant2/1 -> Sum/2
  Constant1/1 -> Product/2
  Math Function1/1 -> Product1/2
  MinMax/1 -> Math Function1/1
  Product/1 -> MinMax/1
  Constant4/1 -> MinMax/2
  Constant3/1 -> Product1/3
  Ncorr (rps)/1 -> Product1/1
  Saturation/1 -> etat (-)/1
  Product1/1 -> Polynomial/1  "BSR"
  Polynomial/1 -> Gain/1
  Gain/1 -> Saturation/1

== system EngineModelsLibrary/Power/Power ==
  W (kg/s) : Inport
  Tin (K) : Inport  Port=2
  Tout (K) : Inport  Port=3
  Constant : Constant  Value=cp
  Product : Product  Inputs=3  RndMeth=Zero
  Sum : Sum  Inputs=|+-
  P (W) : Outport
  wires:
  Tout (K)/1 -> Sum/2
  Tin (K)/1 -> Sum/1
  Constant/1 -> Product/3
  W (kg/s)/1 -> Product/1
  Sum/1 -> Product/2
  Product/1 -> P (W)/1

== system EngineModelsLibrary/Power/Temperature ==
  note: Temperature solved from the definition of efficiency. -- erikhe@umich
  PI (-) : Inport
  Tin (K) : Inport  Port=2
  etat (-) : Inport  Port=3
  Constant1 : Constant  Value=1-1/gam
  Constant2 : Constant
  Divide : Product  Inputs=**
  Divide1 : Product  Inputs=**
  Math Function : Math  Operator=pow  SaturateOnIntegerOverflow=on
  Sum : Sum  Inputs=+-|
  Sum1 : Sum  Inputs=+-|
  Tout (K) : Outport
  wires:
  PI (-)/1 -> Math Function/1
  Constant1/1 -> Math Function/2
  Sum/1 -> Divide/1
  etat (-)/1 -> Divide/2
  Sum1/1 -> Divide1/2
  Tin (K)/1 -> Divide1/1
  Divide1/1 -> Tout (K)/1
  Math Function/1 -> Sum/2
  Constant2/1 -> Sum1/1, Sum/1
  Divide/1 -> Sum1/2

== system EngineModelsLibrary/Small scroll turbine/Mass flow ==
  note: Empirical model of turbine mass flow, see e.g. Eriksson (2007)
      | Modeling and control of turbocharged SI and DI engines, Oil&Gas Science and Technology.
      | Extended by letting the two parameters depend on the mach number ratio r.
      | -- erikhe@umich
  r (-) : Inport
  Pin (Pa) : Inport  Port=2
  Tin (K) : Inport  Port=3
  PI (-) : Inport  Port=4
  Constant1 : Constant  Value=k(3)
  Constant2 : Constant
  Constant3 : Constant  Value=k(4)
  Constant4 : Constant  Value=k(1)
  Constant5 : Constant  Value=0
  Constant6 : Constant  Value=k(2)
  Corrected flow inv : Subsystem
  Gain : Gain  Gain=1e-5
  Math Function : Math  Operator=pow  SaturateOnIntegerOverflow=on
  Math Function1 : Math  Operator=sqrt  SaturateOnIntegerOverflow=on
  MinMax : MinMax  Function=max  Inputs=2
  Product1 : Product  RndMeth=Zero
  Product2 : Product  RndMeth=Zero
  Product3 : Product  RndMeth=Zero
  Saturation : Saturate  UpperLimit=Wclim(2)  LowerLimit=Wclim(1)
  Sum : Sum  Inputs=|-+
  Sum1 : Sum  Inputs=|++
  Sum2 : Sum  Inputs=|++
  Wt (kg/s) : Outport
  wires:
  Product1/1 -> Saturation/1
  Math Function1/1 -> Product1/1
  Tin (K)/1 -> Corrected flow inv/2(Tin (K))
  Pin (Pa)/1 -> Gain/1
  Constant2/1 -> Sum/2
  Math Function/1 -> Sum/1
  PI (-)/1 -> Math Function/1
  Constant5/1 -> MinMax/2
  MinMax/1 -> Math Function1/1
  Sum/1 -> MinMax/1
  Corrected flow inv/1(Wt (kg/s)) -> Wt (kg/s)/1
  Sum1/1 -> Math Function/2
  Constant1/1 -> Sum1/2
  Product3/1 -> Sum1/1
  Constant3/1 -> Product3/2
  r (-)/1 -> Product3/1, Product2/1
  Sum2/1 -> Product1/2
  Constant4/1 -> Sum2/2
  Product2/1 -> Sum2/1
  Constant6/1 -> Product2/2
  Gain/1 -> Corrected flow inv/1(Pin (bar))
  Saturation/1 -> Corrected flow inv/3(Wt corr (kg/s K^.5/bar))

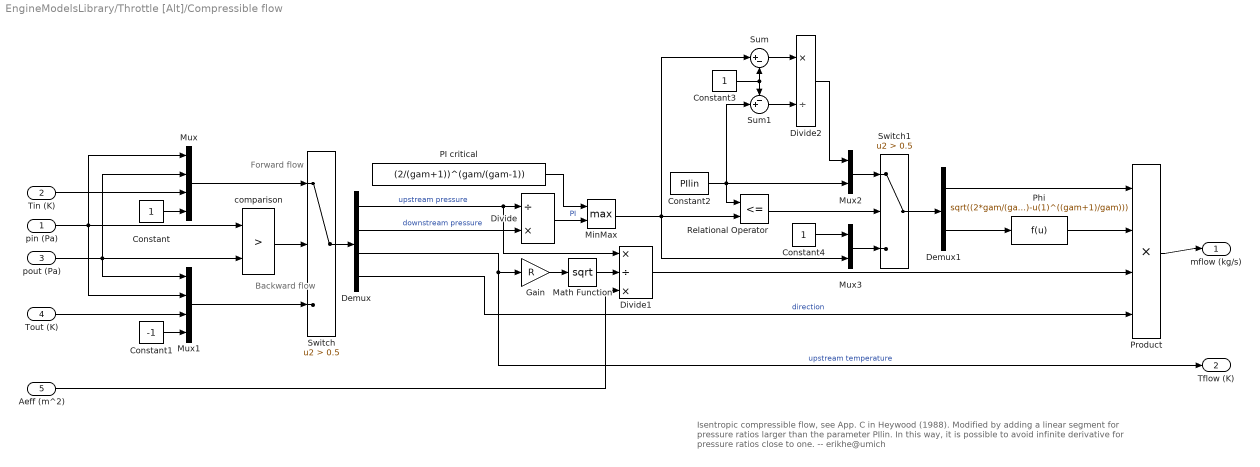
== system EngineModelsLibrary/Throttle [Alt]/Compressible flow ==
  note: Isentropic compressible flow, see App. C in Heywood (1988). Modified by adding a linear segment for pressure ratios larger than
      | the parameter PIlin. In this way, it is possible to avoid infinite derivative for pressure ratios close to one. -- erikhe@umich
  note: Forward flow
  note: Backward flow
  pin (Pa) : Inport
  Tin (K) : Inport  Port=2
  pout (Pa) : Inport  Port=3
  Tout (K) : Inport  Port=4
  Aeff (m^2) : Inport  Port=5
  Constant : Constant
  Constant1 : Constant  Value=-1
  Constant2 : Constant  Value=PIlin
  Constant3 : Constant
  Constant4 : Constant
  Demux : Demux
  Demux1 : Demux  Outputs=2
  Divide : Product  Inputs=/*
  Divide1 : Product  Inputs=*/*
  Divide2 : Product  Inputs=*/
  Gain : Gain  Gain=R
  Math Function : Math  Operator=sqrt  SaturateOnIntegerOverflow=on
  MinMax : MinMax  Function=max  Inputs=2
  Mux : Mux
  Mux1 : Mux
  Mux2 : Mux  Inputs=2
  Mux3 : Mux  Inputs=2
  PI critical : Constant  Value=(2/(gam+1))^(gam/(gam-1))
  Phi : Fcn  Expr=sqrt((2*gam/(gam-1))*(u(1)^(2/gam)-u(1)^((gam+1)/gam)))
  Product : Product  Inputs=4  RndMeth=Zero
  Relational Operator : RelationalOperator  Operator=<=  OutDataTypeStr=boolean
  Sum : Sum  Inputs=|+-
  Sum1 : Sum  Inputs=-+|
  Switch : Switch  Criteria=u2 > Threshold  Threshold=0.5
  Switch1 : Switch  Criteria=u2 > Threshold  Threshold=0.5
  comparison : RelationalOperator  Operator=>  OutDataTypeStr=boolean
  mflow (kg/s) : Outport
  Tflow (K) : Outport  Port=2
  wires:
  Product/1 -> mflow (kg/s)/1
  Divide1/1 -> Product/3
  Demux/4 -> Product/4  "direction"
  Constant1/1 -> Mux1/4
  Constant/1 -> Mux/4
  Math Function/1 -> Divide1/2
  Aeff (m^2)/1 -> Divide1/3
  Gain/1 -> Math Function/1
  PI critical/1 -> MinMax/1
  Demux/3 -> Tflow (K)/1, Gain/1  "upstream temperature"
  Divide/1 -> MinMax/2  "PI"
  Demux/2 -> Divide/2  "downstream pressure"
  Demux/1 -> Divide1/1, Divide/1  "upstream pressure"
  Switch/1 -> Demux/1
  Tout (K)/1 -> Mux1/3
  Tin (K)/1 -> Mux/3
  Mux1/1 -> Switch/3
  Mux/1 -> Switch/1
  pout (Pa)/1 -> Mux1/1, comparison/2, Mux/2
  pin (Pa)/1 -> Mux1/2, comparison/1, Mux/1
  comparison/1 -> Switch/2
  MinMax/1 -> Relational Operator/2, Mux3/2, Sum/1
  Constant2/1 -> Relational Operator/1, Mux2/2, Sum1/2
  Relational Operator/1 -> Switch1/2
  Constant3/1 -> Sum/2, Sum1/1
  Sum/1 -> Divide2/1
  Sum1/1 -> Divide2/2
  Divide2/1 -> Mux2/1
  Mux2/1 -> Switch1/1
  Mux3/1 -> Switch1/3
  Constant4/1 -> Mux3/1
  Switch1/1 -> Demux1/1
  Demux1/2 -> Phi/1
  Demux1/1 -> Product/1
  Phi/1 -> Product/2

== system EngineModelsLibrary/Throttle [Alt]/Throttle area ==
  note: Throttle area. See, e.g., Jiang et al. SAE09010680.
      | -- erikhe@umich
  uth (%) : Inport
  A0 : Constant  Value=Ar0
  A1 : Constant  Value=Ar1
  Constant : Constant
  Constant1 : Constant  Value=b0
  Fcn : Fcn  Expr=(cos(a2*u*u+a1*u+a0))^2
  Gain : Gain  Gain=.01
  Gain1 : Gain  Gain=b1
  Gain2 : Gain  Gain=pi/180
  Product : Product  RndMeth=Zero
  Saturation : Saturate  UpperLimit=100  LowerLimit=0
  Sum : Sum  Inputs=|+-
  Sum1 : Sum  Inputs=|++
  Sum2 : Sum  Inputs=|++
  A (m^2) : Outport
  wires:
  Fcn/1 -> Sum/2
  Gain2/1 -> Fcn/1
  Sum2/1 -> Gain2/1
  Constant1/1 -> Sum2/2
  Gain1/1 -> Sum2/1
  Gain/1 -> Gain1/1
  Saturation/1 -> Gain/1
  Product/1 -> Sum1/1
  Sum/1 -> Product/1
  Sum1/1 -> A (m^2)/1
  A1/1 -> Product/2
  A0/1 -> Sum1/2
  Constant/1 -> Sum/1
  uth (%)/1 -> Saturation/1

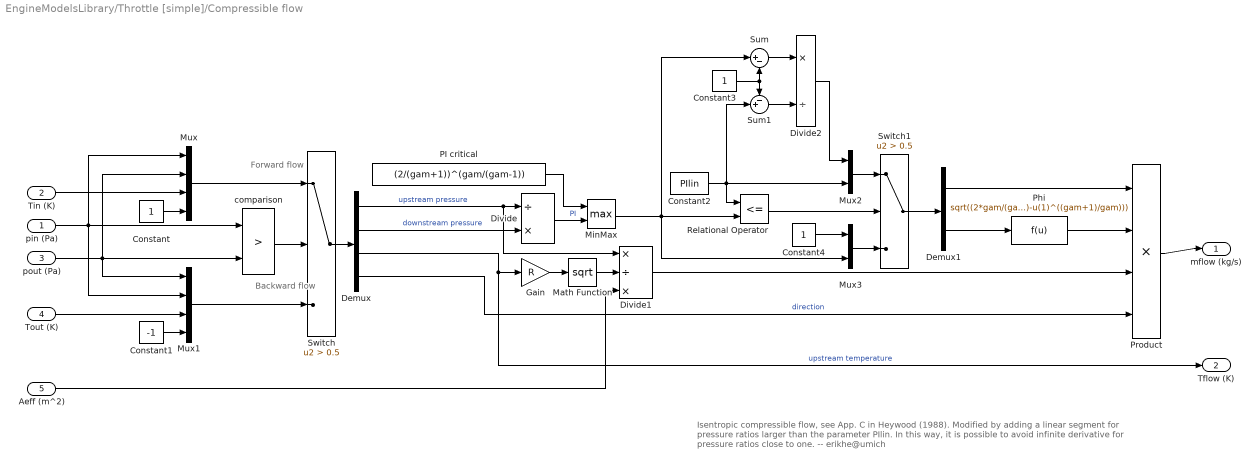
== system EngineModelsLibrary/Throttle [simple]/Compressible flow ==
  note: Backward flow
  note: Forward flow
  note: Isentropic compressible flow, see App. C in Heywood (1988). Modified by adding a linear segment for pressure ratios larger than
      | the parameter PIlin. In this way, it is possible to avoid infinite derivative for pressure ratios close to one. -- erikhe@umich
  pin (Pa) : Inport
  Tin (K) : Inport  Port=2
  pout (Pa) : Inport  Port=3
  Tout (K) : Inport  Port=4
  Aeff (m^2) : Inport  Port=5
  Constant : Constant
  Constant1 : Constant  Value=-1
  Constant2 : Constant  Value=PIlin
  Constant3 : Constant
  Constant4 : Constant
  Demux : Demux
  Demux1 : Demux  Outputs=2
  Divide : Product  Inputs=/*
  Divide1 : Product  Inputs=*/*
  Divide2 : Product  Inputs=*/
  Gain : Gain  Gain=R
  Math Function : Math  Operator=sqrt  SaturateOnIntegerOverflow=on
  MinMax : MinMax  Function=max  Inputs=2
  Mux : Mux
  Mux1 : Mux
  Mux2 : Mux  Inputs=2
  Mux3 : Mux  Inputs=2
  PI critical : Constant  Value=(2/(gam+1))^(gam/(gam-1))
  Phi : Fcn  Expr=sqrt((2*gam/(gam-1))*(u(1)^(2/gam)-u(1)^((gam+1)/gam)))
  Product : Product  Inputs=4  RndMeth=Zero
  Relational Operator : RelationalOperator  Operator=<=  OutDataTypeStr=boolean
  Sum : Sum  Inputs=|+-
  Sum1 : Sum  Inputs=-+|
  Switch : Switch  Criteria=u2 > Threshold  Threshold=0.5
  Switch1 : Switch  Criteria=u2 > Threshold  Threshold=0.5
  comparison : RelationalOperator  Operator=>  OutDataTypeStr=boolean
  mflow (kg/s) : Outport
  Tflow (K) : Outport  Port=2
  wires:
  Phi/1 -> Product/2
  Demux1/1 -> Product/1
  Demux1/2 -> Phi/1
  Switch1/1 -> Demux1/1
  Constant4/1 -> Mux3/1
  Mux3/1 -> Switch1/3
  Mux2/1 -> Switch1/1
  Divide2/1 -> Mux2/1
  Sum1/1 -> Divide2/2
  Sum/1 -> Divide2/1
  Constant3/1 -> Sum1/1, Sum/2
  Relational Operator/1 -> Switch1/2
  Constant2/1 -> Sum1/2, Mux2/2, Relational Operator/1
  MinMax/1 -> Sum/1, Mux3/2, Relational Operator/2
  comparison/1 -> Switch/2
  pin (Pa)/1 -> Mux/1, comparison/1, Mux1/2
  pout (Pa)/1 -> Mux/2, comparison/2, Mux1/1
  Mux/1 -> Switch/1
  Mux1/1 -> Switch/3
  Tin (K)/1 -> Mux/3
  Tout (K)/1 -> Mux1/3
  Switch/1 -> Demux/1
  Demux/1 -> Divide/1, Divide1/1  "upstream pressure"
  Demux/2 -> Divide/2  "downstream pressure"
  Divide/1 -> MinMax/2  "PI"
  Demux/3 -> Gain/1, Tflow (K)/1  "upstream temperature"
  PI critical/1 -> MinMax/1
  Gain/1 -> Math Function/1
  Aeff (m^2)/1 -> Divide1/3
  Math Function/1 -> Divide1/2
  Constant/1 -> Mux/4
  Constant1/1 -> Mux1/4
  Demux/4 -> Product/4  "direction"
  Divide1/1 -> Product/3
  Product/1 -> mflow (kg/s)/1

== system EngineModelsLibrary/Throttle [simple]/Throttle area ==
  alpha (rad) : Inport
  Constant : Constant
  Maximum Area : Constant  Value=Amax
  Minimum Area : Constant  Value=Amin
  Product : Product  RndMeth=Zero
  Saturation : Saturate  UpperLimit=pi  LowerLimit=0
  Sum : Sum  Inputs=|+-
  Sum1 : Sum  Inputs=|++
  Sum2 : Sum  Inputs=|+-
  Trigonometric Function : Trigonometry  Operator=cos
  A (m^2) : Outport
  wires:
  alpha (rad)/1 -> Saturation/1
  Saturation/1 -> Trigonometric Function/1
  Constant/1 -> Sum/1
  Trigonometric Function/1 -> Sum/2
  Minimum Area/1 -> Sum1/2, Sum2/2
  Maximum Area/1 -> Sum2/1
  Sum1/1 -> A (m^2)/1
  Sum/1 -> Product/1
  Product/1 -> Sum1/1
  Sum2/1 -> Product/2

== system EngineModelsLibrary/Turbine [Eriksson]/Efficiency ==
  note: Empirical model of turbine efficiency, see e.g. Eriksson (2007)
      | Modeling and control of turbocharged SI and DI engines, Oil&Gas Science and Technology. -- erikhe@umich
  PI (-) : Inport
  Tin (K) : Inport  Port=2
  w (rad/s) : Inport  Port=3
  Constant : Constant  Value=1-1/gam
  Constant1 : Constant  Value=2*cp
  Constant2 : Constant
  Constant3 : Constant  Value=D/2
  Constant4 : Constant  Value=eps
  Constant5 : Constant  Value=BSRmax
  Constant6 : Constant
  Gain : Gain  Gain=ct
  Gain1 : Gain  Gain=etamax
  Math Function : Math  Operator=pow  SaturateOnIntegerOverflow=on
  Math Function1 : Math  Operator=sqrt  SaturateOnIntegerOverflow=on
  Math Function2 : Math  Operator=square  SaturateOnIntegerOverflow=on
  MinMax : MinMax  Function=max  Inputs=2
  Product : Product  Inputs=3  RndMeth=Zero
  Product1 : Product  Inputs=*/*  RndMeth=Zero
  Saturation : Saturate  UpperLimit=etamax  LowerLimit=etamin
  Sum : Sum  Inputs=|-+
  Sum1 : Sum  Inputs=|+-
  Sum2 : Sum  Inputs=|-+
  etat (-) : Outport
  wires:
  Constant/1 -> Math Function/2
  PI (-)/1 -> Math Function/1
  Math Function/1 -> Sum/1
  Constant2/1 -> Sum/2
  Sum/1 -> Product/2
  Constant1/1 -> Product/3
  Tin (K)/1 -> Product/1
  Math Function1/1 -> Product1/2
  MinMax/1 -> Math Function1/1
  Product/1 -> MinMax/1
  Constant4/1 -> MinMax/2
  Constant3/1 -> Product1/3
  w (rad/s)/1 -> Product1/1
  Product1/1 -> Sum1/1  "BSR"
  Constant5/1 -> Sum1/2
  Sum1/1 -> Math Function2/1
  Math Function2/1 -> Gain/1
  Constant6/1 -> Sum2/2
  Gain/1 -> Sum2/1
  Sum2/1 -> Gain1/1
  Gain1/1 -> Saturation/1
  Saturation/1 -> etat (-)/1

== system EngineModelsLibrary/Turbine [Eriksson]/Mass flow ==
  note: Empirical model of turbine mass flow, see e.g. Eriksson (2007)
      | Modeling and control of turbocharged SI and DI engines, Oil&Gas Science and Technology. -- erikhe@umich
  pin (Pa) : Inport
  Tin (K) : Inport  Port=2
  PI (-) : Inport  Port=3
  Constant1 : Constant  Value=k1
  Constant2 : Constant
  Constant5 : Constant  Value=0
  Corrected flow inv : Subsystem
  Gain : Gain  Gain=k0
  Math Function : Math  Operator=pow  SaturateOnIntegerOverflow=on
  Math Function1 : Math  Operator=sqrt  SaturateOnIntegerOverflow=on
  MinMax : MinMax  Function=max  Inputs=2
  Sum : Sum  Inputs=|-+
  Wt (kg/s) : Outport
  wires:
  Gain/1 -> Corrected flow inv/3(Wcorr (kg/s))
  Math Function1/1 -> Gain/1
  Tin (K)/1 -> Corrected flow inv/2(Tin (K))
  pin (Pa)/1 -> Corrected flow inv/1(pin (Pa))
  Constant2/1 -> Sum/2
  Math Function/1 -> Sum/1
  Constant1/1 -> Math Function/2
  PI (-)/1 -> Math Function/1
  Constant5/1 -> MinMax/2
  MinMax/1 -> Math Function1/1
  Sum/1 -> MinMax/1
  Corrected flow inv/1(W (kg/s)) -> Wt (kg/s)/1

== system EngineModelsLibrary/Turbine [Eriksson]/Power ==
  W (kg/s) : Inport
  Tin (K) : Inport  Port=2
  Tout (K) : Inport  Port=3
  Constant : Constant  Value=cp
  Product : Product  Inputs=3  RndMeth=Zero
  Sum : Sum  Inputs=|+-
  P (W) : Outport
  wires:
  Product/1 -> P (W)/1
  Sum/1 -> Product/2
  W (kg/s)/1 -> Product/1
  Constant/1 -> Product/3
  Tin (K)/1 -> Sum/1
  Tout (K)/1 -> Sum/2

== system EngineModelsLibrary/Turbine [Eriksson]/Pressure ratio w saturation ==
  pin (Pa) : Inport
  pout (Pa) : Inport  Port=2
  Constant : Constant
  Divide : Product  Inputs=*/
  MinMax : MinMax  Inputs=2
  PI (-) : Outport
  wires:
  MinMax/1 -> PI (-)/1
  Constant/1 -> MinMax/2
  Divide/1 -> MinMax/1
  pin (Pa)/1 -> Divide/2
  pout (Pa)/1 -> Divide/1

== system EngineModelsLibrary/Turbine [Eriksson]/Temperature ==
  note: Temperature solved from the definition of efficiency. -- erikhe@umich
  PI (-) : Inport
  Tin (K) : Inport  Port=2
  etat (-) : Inport  Port=3
  Constant1 : Constant  Value=1-1/gam
  Constant2 : Constant
  Divide : Product  Inputs=**
  Divide1 : Product  Inputs=**
  Math Function : Math  Operator=pow  SaturateOnIntegerOverflow=on
  Sum : Sum  Inputs=+-|
  Sum1 : Sum  Inputs=+-|
  Tout (K) : Outport
  wires:
  Divide/1 -> Sum1/2
  Constant2/1 -> Sum/1, Sum1/1
  Math Function/1 -> Sum/2
  Divide1/1 -> Tout (K)/1
  Tin (K)/1 -> Divide1/1
  Sum1/1 -> Divide1/2
  etat (-)/1 -> Divide/2
  Sum/1 -> Divide/1
  Constant1/1 -> Math Function/2
  PI (-)/1 -> Math Function/1

== system EngineModelsLibrary/Turbine [Jensen,Moraal]/Corrected speed ==
  note: Speed corrected based on inlet conditions.
      | -- erikhe@umich
  Tin (K) : Inport
  w (rad/s) : Inport  Port=2
  Divide1 : Product  Inputs=*/
  Gain : Gain  Gain=1/(2*pi)
  Math Function : Math  Operator=sqrt  SaturateOnIntegerOverflow=on
  Nc corr (rps/K^.5) : Outport
  wires:
  Tin (K)/1 -> Math Function/1
  w (rad/s)/1 -> Gain/1
  Math Function/1 -> Divide1/2
  Divide1/1 -> Nc corr (rps/K^.5)/1
  Gain/1 -> Divide1/1
